simulink subsystem "hexa_groundcontact_forces_moments"  (R2024a)
settings: Solver=VariableStepAuto  StartTime=0.0  StopTime=10.0  RelTol=1e-3
undefined symbols (not defined in the file or in its folder): contact, control
libraries: simulink x1
settings Model: Creator=user  LastModifiedBy=user

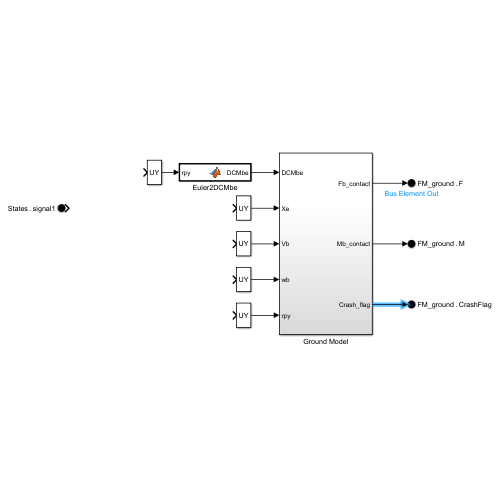
[thumbnail: Simulink's stored preview of the top-level diagram]
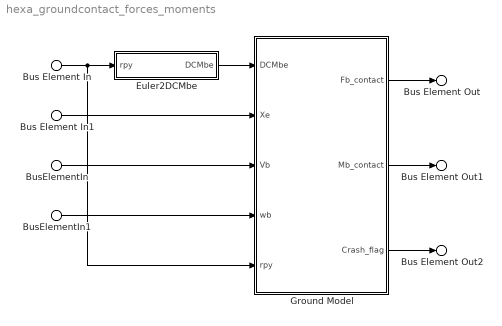
== system hexa_groundcontact_forces_moments ==
  Bus Element In : Inport  PortName=States  Element=Euler
  Bus Element In1 : Inport  PortName=States  Element=XYZ
  BusElementIn : Inport  PortName=States  Element=UVWb
  BusElementIn1 : Inport  PortName=States  Element=PQR
  Euler2DCMbe : MATLAB Function  TreatAsAtomicUnit=on
  Ground Model : Subsystem
  Bus Element Out : Outport  PortName=FM_groundcontact  Element=Fb
  Bus Element Out1 : Outport  PortName=FM_groundcontact  Element=Mb
  Bus Element Out2 : Outport  PortName=FM_groundcontact  Element=CrashFlag
  wires:
  Bus Element In/1 -> Euler2DCMbe/1(rpy), Ground Model/5(rpy)
  BusElementIn1/1 -> Ground Model/4(wb)
  Ground Model/3(Crash_flag) -> Bus Element Out2/1
  BusElementIn/1 -> Ground Model/3(Vb)
  Ground Model/1(Fb_contact) -> Bus Element Out/1
  Bus Element In1/1 -> Ground Model/2(Xe)
  Euler2DCMbe/1(DCMbe) -> Ground Model/1(DCMbe)
  Ground Model/2(Mb_contact) -> Bus Element Out1/1

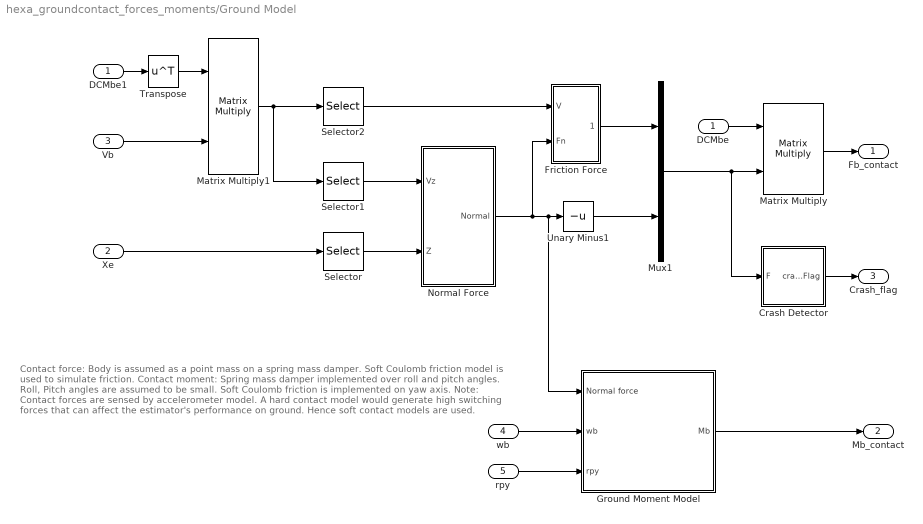
== system hexa_groundcontact_forces_moments/Ground Model ==
  note: Contact force:
      | Body is assumed as a point mass on a spring mass damper. Soft Coulomb friction model is used to simulate friction.
      |
      | Contact moment:
      | Spring mass damper implemented over roll and pitch angles. Roll, Pitch angles are assumed to be small.
      | Soft Coulomb friction is implemented on yaw axis.
      |
      | Note:
      | Contact forces are sensed by accelerometer model. A hard contact model would generate high switching forces that can affect the estimator's performance on ground. Hence soft contact models are used.
  DCMbe : Inport
  Xe : Inport  Port=2
  Vb : Inport  Port=3
  wb : Inport  Port=4
  rpy : Inport  Port=5
  Crash Detector : Subsystem
  DCMbe1 : InportShadow
  Friction Force : Subsystem
  Ground Moment Model : Subsystem
  Matrix Multiply : Product  Multiplication=Matrix(*)
  Matrix Multiply1 : Product  Multiplication=Matrix(*)
  Mux1 : Mux  Inputs=2
  Normal Force : Subsystem
  Selector : Selector  InputPortWidth=3  IndexOptions=Index vector (dialog)  Indices=[3]  OutputSizes=1
  Selector1 : Selector  InputPortWidth=3  IndexOptions=Index vector (dialog)  Indices=[3]  OutputSizes=1
  Selector2 : Selector  InputPortWidth=3  IndexOptions=Index vector (dialog)  Indices=[1,2]  OutputSizes=1
  Transpose : Math  Operator=transpose
  Unary Minus1 : UnaryMinus
  Fb_contact : Outport
  Mb_contact : Outport  Port=2
  Crash_flag : Outport  Port=3
  wires:
  Ground Moment Model/1(Mb) -> Mb_contact/1
  rpy/1 -> Ground Moment Model/3(rpy)
  wb/1 -> Ground Moment Model/2(wb)
  Matrix Multiply1/1 -> Selector2/1, Selector1/1
  Vb/1 -> Matrix Multiply1/2
  Transpose/1 -> Matrix Multiply1/1
  DCMbe1/1 -> Transpose/1
  Friction Force/1(Friction) -> Mux1/1
  Selector2/1 -> Friction Force/1(V)
  Unary Minus1/1 -> Mux1/2
  Mux1/1 -> Matrix Multiply/2, Crash Detector/1(F)
  Normal Force/1(Normal) -> Friction Force/2(Fn), Unary Minus1/1, Ground Moment Model/1(Normal force)
  Matrix Multiply/1 -> Fb_contact/1
  DCMbe/1 -> Matrix Multiply/1
  Selector/1 -> Normal Force/2(Z)
  Selector1/1 -> Normal Force/1(Vz)
  Xe/1 -> Selector/1
  Crash Detector/1(crashFlag) -> Crash_flag/1

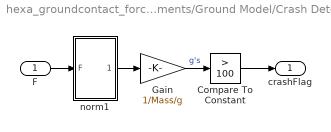
== system hexa_groundcontact_forces_moments/Ground Model/Crash Detector ==
  F : Inport
  Compare To Constant : simulink/Logic and Bit Operations/Compare To Constant  relop=>  const=100  OutDataTypeStr=boolean
  Gain : Gain  Gain=1/Mass/g
  norm1 : Subsystem
  crashFlag : Outport
  wires:
  Gain/1 -> Compare To Constant/1  "g's"
  Compare To Constant/1 -> crashFlag/1
  norm1/1(Out1) -> Gain/1
  F/1 -> norm1/1(F)

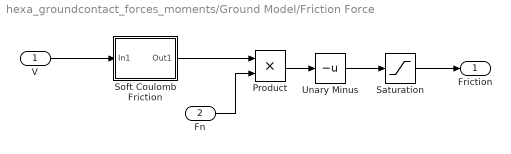
== system hexa_groundcontact_forces_moments/Ground Model/Friction Force ==
  V : Inport
  Fn : Inport  Port=2
  Product : Product
  Saturation : Saturate  UpperLimit=contact.translation.maxFriction  LowerLimit=-contact.translation.maxFriction
  Soft Coulomb Friction : Subsystem
  Unary Minus : UnaryMinus
  Friction : Outport
  wires:
  Saturation/1 -> Friction/1
  Unary Minus/1 -> Saturation/1
  V/1 -> Soft Coulomb Friction/1(In1)
  Product/1 -> Unary Minus/1
  Soft Coulomb Friction/1(Out1) -> Product/1
  Fn/1 -> Product/2

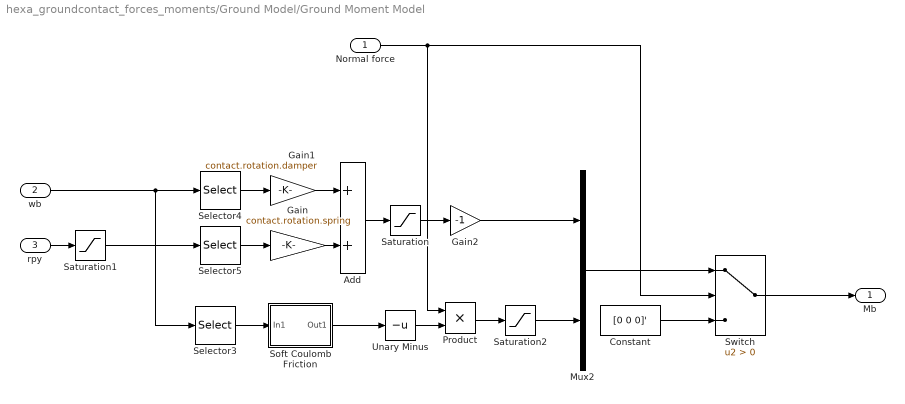
== system hexa_groundcontact_forces_moments/Ground Model/Ground Moment Model ==
  Normal force : Inport
  wb : Inport  Port=2
  rpy : Inport  Port=3
  Add : Sum
  Constant : Constant  Value=[0 0 0]'
  Gain : Gain  Gain=contact.rotation.spring
  Gain1 : Gain  Gain=contact.rotation.damper
  Gain2 : Gain  Gain=-1
  Mux2 : Mux  Inputs=2
  Product : Product
  Saturation : Saturate  UpperLimit=control.rotation.maxMoment  LowerLimit=-control.rotation.maxMoment
  Saturation1 : Saturate  UpperLimit=20*pi/180  LowerLimit=-20*pi/180
  Saturation2 : Saturate  UpperLimit=control.rotation.maxMoment  LowerLimit=-control.rotation.maxMoment
  Selector3 : Selector  InputPortWidth=3  IndexOptions=Index vector (dialog)  Indices=[3]  OutputSizes=1
  Selector4 : Selector  InputPortWidth=3  IndexOptions=Index vector (dialog)  Indices=[1, 2]  OutputSizes=1
  Selector5 : Selector  InputPortWidth=3  IndexOptions=Index vector (dialog)  Indices=[1, 2]  OutputSizes=1
  Soft Coulomb Friction : Subsystem
  Switch : Switch  Criteria=u2 > Threshold  SaturateOnIntegerOverflow=off  InputSameDT=off
  Unary Minus : UnaryMinus
  Mb : Outport
  wires:
  Saturation2/1 -> Mux2/2
  Product/1 -> Saturation2/1
  Unary Minus/1 -> Product/2
  Soft Coulomb Friction/1(Out1) -> Unary Minus/1
  Selector3/1 -> Soft Coulomb Friction/1(In1)
  wb/1 -> Selector3/1, Selector4/1
  Saturation1/1 -> Selector5/1
  rpy/1 -> Saturation1/1
  Normal force/1 -> Switch/2, Product/1
  Mux2/1 -> Switch/1
  Switch/1 -> Mb/1
  Selector5/1 -> Gain/1
  Constant/1 -> Switch/3
  Gain1/1 -> Add/1
  Selector4/1 -> Gain1/1
  Saturation/1 -> Gain2/1
  Gain/1 -> Add/2
  Add/1 -> Saturation/1
  Gain2/1 -> Mux2/1

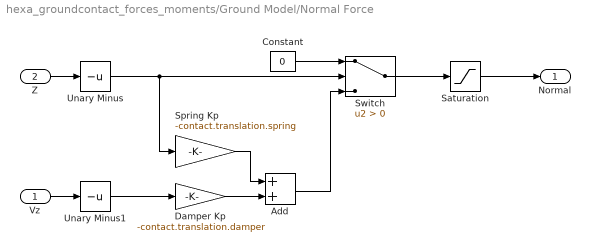
== system hexa_groundcontact_forces_moments/Ground Model/Normal Force ==
  Vz : Inport
  Z : Inport  Port=2
  Add : Sum
  Constant : Constant  Value=0
  Damper Kp : Gain  Gain=-contact.translation.damper
  Saturation : Saturate  UpperLimit=contact.translation.maxNormal  LowerLimit=0
  Spring Kp : Gain  Gain=-contact.translation.spring
  Switch : Switch  Criteria=u2 > Threshold  SaturateOnIntegerOverflow=off  InputSameDT=off
  Unary Minus : UnaryMinus
  Unary Minus1 : UnaryMinus
  Normal : Outport
  wires:
  Unary Minus1/1 -> Damper Kp/1
  Unary Minus/1 -> Switch/2, Spring Kp/1
  Saturation/1 -> Normal/1
  Vz/1 -> Unary Minus1/1
  Spring Kp/1 -> Add/1
  Add/1 -> Switch/3
  Damper Kp/1 -> Add/2
  Switch/1 -> Saturation/1
  Z/1 -> Unary Minus/1
  Constant/1 -> Switch/1

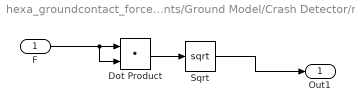
== system hexa_groundcontact_forces_moments/Ground Model/Crash Detector/norm1 ==
  F : Inport
  Dot Product : DotProduct  OutDataTypeStr=Inherit: Inherit via internal rule
  Sqrt : Sqrt
  Out1 : Outport
  wires:
  Sqrt/1 -> Out1/1
  F/1 -> Dot Product/1, Dot Product/2
  Dot Product/1 -> Sqrt/1

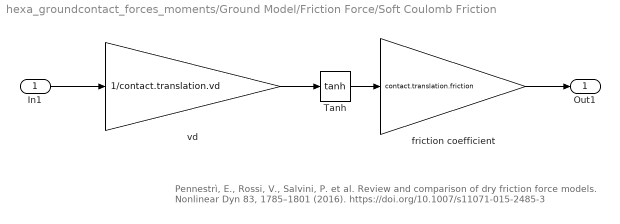
== system hexa_groundcontact_forces_moments/Ground Model/Friction Force/Soft Coulomb Friction ==
  note: Pennestrì, E., Rossi, V., Salvini, P. et al. Review and comparison of dry friction force models. Nonlinear Dyn 83, 1785–1801 (2016). https://doi.org/10.1007/s11071-015-2485-3
  In1 : Inport
  Tanh : Trigonometry  Operator=tanh
  friction coefficient : Gain  Gain=contact.translation.friction
  vd : Gain  Gain=1/contact.translation.vd
  Out1 : Outport
  wires:
  friction coefficient/1 -> Out1/1
  Tanh/1 -> friction coefficient/1
  vd/1 -> Tanh/1
  In1/1 -> vd/1

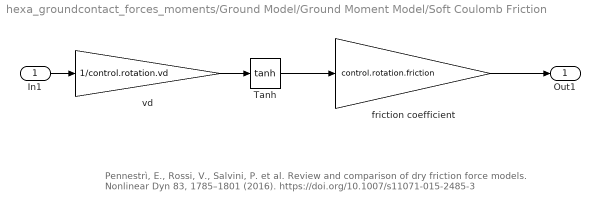
== system hexa_groundcontact_forces_moments/Ground Model/Ground Moment Model/Soft Coulomb Friction ==
  note: Pennestrì, E., Rossi, V., Salvini, P. et al. Review and comparison of dry friction force models. Nonlinear Dyn 83, 1785–1801 (2016). https://doi.org/10.1007/s11071-015-2485-3
  In1 : Inport
  Tanh : Trigonometry  Operator=tanh
  friction coefficient : Gain  Gain=control.rotation.friction
  vd : Gain  Gain=1/control.rotation.vd
  Out1 : Outport
  wires:
  friction coefficient/1 -> Out1/1
  Tanh/1 -> friction coefficient/1
  vd/1 -> Tanh/1
  In1/1 -> vd/1

== matlab function hexa_groundcontact_forces_moments/Euler2DCMbe ==
  data: rpy input; DCMbe output
function DCMbe = fcn(rpy)

phi = rpy(1); theta = rpy(2); psi = rpy(3);
DCMbe = [ cos(psi)*cos(theta), sin(psi)*cos(theta), -sin(theta);
      -sin(psi)*cos(phi)+cos(psi)*sin(theta)*sin(phi), cos(psi)*cos(phi)+sin(psi)*sin(theta)*sin(phi), cos(theta)*sin(phi);
      sin(psi)*sin(phi)+cos(psi)*sin(theta)*cos(phi), -cos(psi)*sin(phi)+sin(psi)*sin(theta)*cos(phi), cos(theta)*cos(phi);
];
